simulink model "sol5_cubic_disturbance"  (R2021b)
settings: Solver=VariableStepAuto  StartTime=0.0  StopTime=1.5  RelTol=1e-3
PreLoadFcn:
  | initModelData
  | trajectoryData
  | controlPD
StartFcn:
  | controlPD
values from neighbouring files (symbols this model uses):
  B = Bm+(Kb*Km/R)    (= 0.0149065789474)    [MyData_for_1_and_2.m]    (also in MyData_for_3_4_and_5.m; MyData_for_5_and_6.m)
  Jm = 5.5e-4    (= 0.00055)    [MyData_for_1_and_2.m]    (also in MyData_for_3_4_and_5.m; MyData_for_5_and_6.m)
  Kd = (R/Km)*((2*Jm*w*zeta)-B)    (= 0.369819047619)    [MyData_for_1_and_2.m]    (also in MyData_for_3_4_and_5.m = 0.2902; MyData_for_5_and_6.m = 0.0513428571429)
  Km = 0.105    [MyData_for_1_and_2.m]    (also in MyData_for_3_4_and_5.m; MyData_for_5_and_6.m)
  Kp = (R/Km)*(Jm*(w^2))    (= 14.3314285714)    [MyData_for_1_and_2.m]    (also in MyData_for_3_4_and_5.m = 9.95238095238; MyData_for_5_and_6.m = 1.59238095238)
  R = 0.76    [MyData_for_1_and_2.m]    (also in MyData_for_3_4_and_5.m; MyData_for_5_and_6.m)
  r = 156    [MyData_for_1_and_2.m]    (also in MyData_for_3_4_and_5.m; MyData_for_5_and_6.m)
settings Model: Creator=esdan  LastModifiedBy=munir
settings SolverCC: AlgebraicLoopSolver=TrustRegion
settings DebuggingCC: SFMachineParentedDataDiag=warning

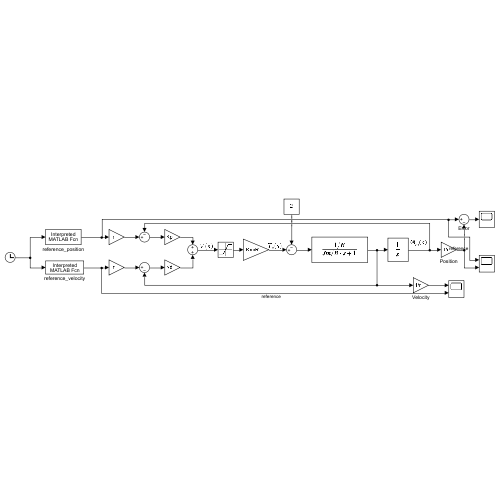
[thumbnail: Simulink's stored preview of the top-level diagram]
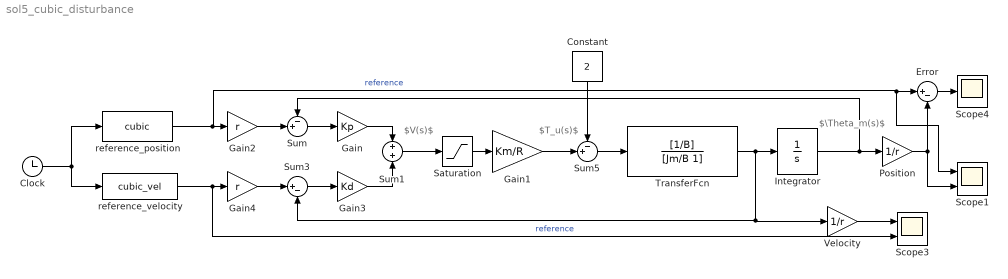
== system sol5_cubic_disturbance ==
  note: $\Theta_m(s)$
  note: $V(s)$
  note: $T_u(s)$
  Clock : Clock
  Constant : Constant  Value=2
  Error : Sum  Inputs=|+-
  Gain : Gain  Gain=Kp
  Gain1 : Gain  Gain=Km/R
  Gain2 : Gain  Gain=r
  Gain3 : Gain  Gain=Kd
  Gain4 : Gain  Gain=r
  Integrator : Integrator
  Position : Gain  Gain=1/r
  Saturation : Saturate  UpperLimit=35  LowerLimit=-35
  Scope1 : Scope  NumInputPorts=2
  Scope3 : Scope  NumInputPorts=2
  Scope4 : Scope
  Sum : Sum  Inputs=-+|
  Sum1 : Sum  Inputs=+|+
  Sum3 : Sum  Inputs=|+-
  Sum5 : Sum  Inputs=-+|
  TransferFcn : TransferFcn  Numerator=[1/B]  Denominator=[Jm/B 1]
  Velocity : Gain  Gain=1/r
  reference_position : MATLABFcn  MATLABFcn=cubic
  reference_velocity : MATLABFcn  MATLABFcn=cubic_vel
  wires:
  TransferFcn/1 -> Integrator/1, Velocity/1, Sum3/2
  Saturation/1 -> Gain1/1
  Sum/1 -> Gain/1
  Gain/1 -> Sum1/1
  Sum1/1 -> Saturation/1
  Gain2/1 -> Sum/2
  reference_position/1 -> Scope1/1, Error/1, Gain2/1  "reference"
  Error/1 -> Scope4/1
  Gain3/1 -> Sum1/2
  Sum3/1 -> Gain3/1
  Position/1 -> Scope1/2, Error/2
  Integrator/1 -> Position/1, Sum/1
  reference_velocity/1 -> Scope3/2, Gain4/1  "reference"
  Gain4/1 -> Sum3/1
  Velocity/1 -> Scope3/1
  Sum5/1 -> TransferFcn/1
  Gain1/1 -> Sum5/2
  Constant/1 -> Sum5/1
  Clock/1 -> reference_velocity/1, reference_position/1
